simulink model "Boost_Converter_v2"  (Simulink 8.5)
settings: Solver=ode23tb  StartTime=0.0  StopTime=1  MaxStep=1e-5  RelTol=1e-9
libraries: powerlib x12, simulink x1
settings Model: Creator=Shailesh  LastModifiedBy=tesla
settings SolverCC: MaxConsecutiveMinStep=20
settings OptimizationCC: InitFltsAndDblsToZero=on
settings DebuggingCC: SaveWithParameterizedLinksMsg=none  SignalResolutionControl=TryResolveAllWithWarning  SolverPrmCheckMsg=warning  MultiTaskDSMMsg=warning  MultiTaskCondExecSysMsg=none  FcnCallInpInsideContextMsg=UseLocalSettings
settings GRTTargetCC: TargetFcnLib=ansi_tfl_tmw.mat

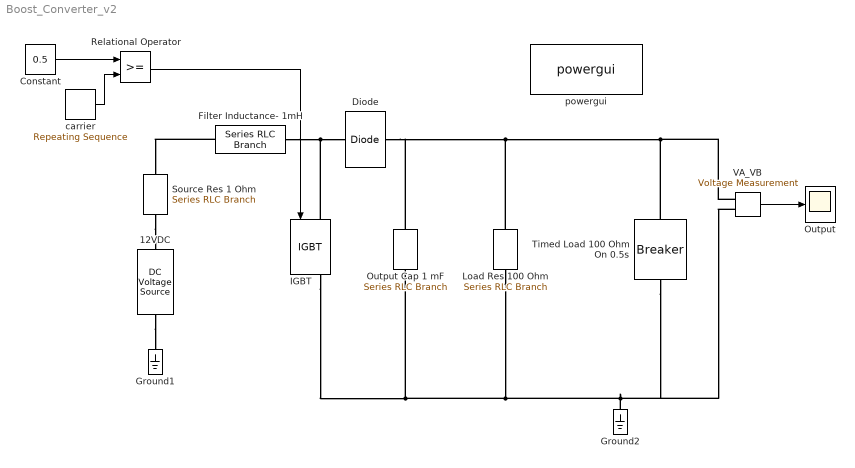
== system Boost_Converter_v2 ==
  12VDC : powerlib/Electrical Sources/DC Voltage Source  Amplitude=12  Measurements=None
  Constant : Constant  Value=0.5
  Diode : powerlib/Power Electronics/Diode  Ron=1e-3  Lon=0  Vf=1  IC=0  UseSnubber=off  Rs=0  Cs=0  Measurements=off
  Filter Inductance- 1mH : powerlib/Elements/Series RLC Branch  LConnTagsString=__new0  RConnTagsString=__new0  BranchType=RL  Resistance=300e-3  Inductance=1e-3  SetiL0=off  InitialCurrent=0  Capacitance=inf  Setx0=off  InitialVoltage=0  Measurements=None
  Ground1 : powerlib/Elements/Ground  LConnTagsString=a
  Ground2 : powerlib/Elements/Ground  LConnTagsString=a
  IGBT : powerlib/Power Electronics/IGBT  Ron=.286e-3  Lon=0  Vf=1  Tf=1e-6  Tt=300e-9  IC=0  Rs=10000  Cs=1e-6  Measurements=on
  Load Res 100 Ohm : powerlib/Elements/Series RLC Branch  LConnTagsString=__new0  RConnTagsString=__new0  BranchType=R  Resistance=100  Inductance=.2  SetiL0=off  InitialCurrent=0  Capacitance=10e-3  Setx0=off  InitialVoltage=600  Measurements=None
  Output : Scope
      settings: YMin=17.6  YMax=19.4  MaxDataPoints=5000000
  Output Cap 1 mF : powerlib/Elements/Series RLC Branch  LConnTagsString=__new0  RConnTagsString=__new0  BranchType=C  Resistance=1  Inductance=.2  SetiL0=off  InitialCurrent=0  Capacitance=1e-3  Setx0=off  InitialVoltage=600  Measurements=None
  Relational Operator : RelationalOperator  OutDataTypeStr=boolean  ZeroCross=off
  Source Res 1 Ohm : powerlib/Elements/Series RLC Branch  LConnTagsString=__new0  RConnTagsString=__new0  BranchType=R  Resistance=1  Inductance=.2  SetiL0=off  InitialCurrent=0  Capacitance=10e-3  Setx0=off  InitialVoltage=600  Measurements=None
  Timed Load 100 Ohm On 0.5s : powerlib/Elements/Breaker  InitialState=0  SwitchingTimes=[0.5]  External=off  BreakerResistance=100  SnubberResistance=1e6  SnubberCapacitance=inf  Measurements=None  MoreParameters=on  NoBreakLoop=off
  VA_VB : powerlib/Measurements/Voltage Measurement  PhasorSimulation=off  OutputType=Complex  PSBequivalent=0
  carrier : simulink/Sources/Repeating Sequence  rep_seq_t=[0 1/20e3]  rep_seq_y=[0 1]
  powergui : powerlib/powergui  Priority=1  SimulationMode=Continuous  SolverType=Tustin  SampleTime=50e-7  frequency=60  SPID=off  DisableSnubberDevices=off  DisableRonSwitches=off  DisableVfSwitches=off  SwTol=0  DisplayEquations=off  Interpol=off  methode=off  Ts=0  FunctionMessages=off  echomessages=off  HookPort=off  EnableUseOfTLC=off  x0status=blocks  frequencyindice=0  Pbase=100e6  ErrMax=1e-4  Iterations=50  UnitsV=kV  UnitsW=MW  buscounter=0  RestoreLinks=warning  ResistiveCurrentMeasurement=off  Frange=[0:2:500]  Ylog=off  Xlog=on  ShowGrid=off  save=off  variable=ZData  structure=0  ZoomFFT=off  StartTime=0.0  cycles=1  DisplayStyle=1  fundamental=60  FreqAxis=off  MaxFrequency=1000  frequencyindicesteady=1  RmsSteady=1  display=off
  wires:
  carrier/1 -> Relational Operator/2
  VA_VB/1 -> Output/1
  Constant/1 -> Relational Operator/1
  Relational Operator/1 -> IGBT/1
  connections:
  12VDC/LConn1 -- Ground1/LConn1
  Timed Load 100 Ohm On 0.5s/LConn1 -- Output Cap 1 mF/LConn1 -- Diode/RConn1 -- Load Res 100 Ohm/LConn1 -- VA_VB/LConn1
  Load Res 100 Ohm/RConn1 -- Timed Load 100 Ohm On 0.5s/RConn1 -- VA_VB/LConn2 -- Ground2/LConn1 -- IGBT/RConn1 -- Output Cap 1 mF/RConn1
  Source Res 1 Ohm/RConn1 -- 12VDC/RConn1
  IGBT/LConn1 -- Filter Inductance- 1mH/RConn1 -- Diode/LConn1
  Filter Inductance- 1mH/LConn1 -- Source Res 1 Ohm/LConn1
